simulink model "model_min_mine"  (R2018a)
settings: Solver=ode45  StartTime=0.0  StopTime=20  RelTol=1e-3
(part 1 of 10)
settings Model: Creator=Роман Стукан  LastModifiedBy=Роман Стукан

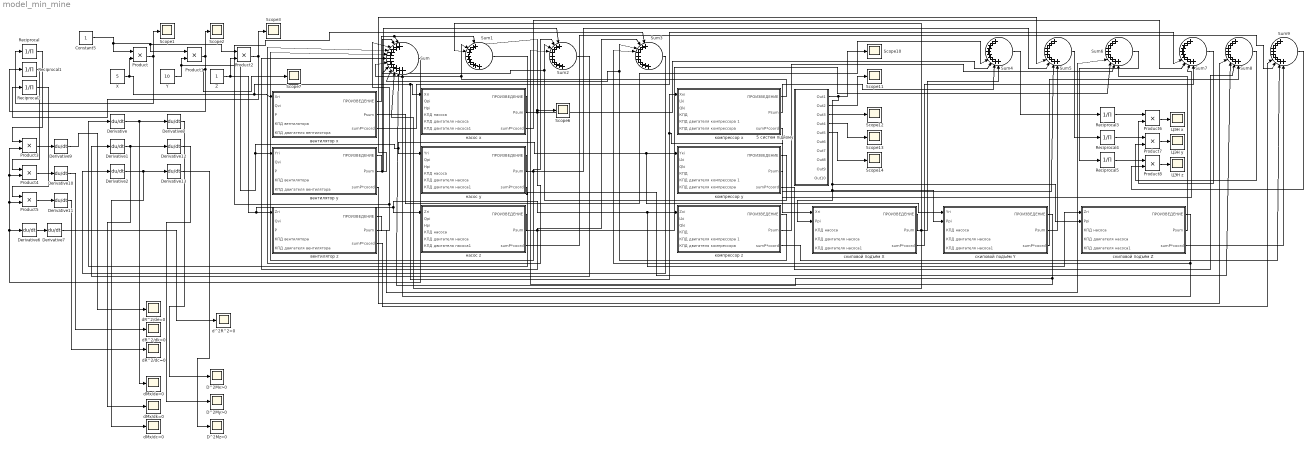
== system model_min_mine ==
  5 систем підйому : Subsystem
  Constant5 : Constant
  D^2Mx>0 : Scope
  D^2My>0 : Scope
  D^2Mz>0 : Scope
  Derivative{,1..2,6..13} (11 alike) : Derivative
  Product{,1..8} (9 alike) : Product
  Reciprocal{,1..5} (6 alike) : Product  Inputs=/  SaturateOnIntegerOverflow=on  RndMeth=Zero
  Scope{1..3,6..7,10..14} (10 alike) : Scope
  Sum : Sum  Inputs=|++++++++++++
  Sum{1..9} (9 alike) : Sum  Inputs=|++++++++++
  X : Constant  Value=5
  Y : Constant  Value=10
  Z : Constant
  dMx/dc=0 : Scope
  dMx/de=0 : Scope
  dMx/dk=0 : Scope
  dR^2/dc=0 : Scope
  dR^2/de=0 : Scope
  dR^2/dk=0 : Scope
  d^2R^2>0 : Scope
  ЦЭН x : Scope
  ЦЭН y : Scope
  ЦЭН z : Scope
  вентилятор x : Subsystem
  вентилятор y : Subsystem
  вентилятор z : Subsystem
  компрессор x : Subsystem
  компрессор y : Subsystem
  компрессор z : Subsystem
  насос x : Subsystem
  насос y : Subsystem
  насос z : Subsystem
  скиповой подъём Y : Subsystem
  скиповой подъём Z : Subsystem
  скиповой подъём Х : Subsystem
  wires:
  X/1 -> Product/2, скиповой подъём Х/1(Xri), компрессор x/1(Xкi), насос x/1(Xri), вентилятор x/1(Xri)
  Y/1 -> Product1/2, скиповой подъём Y/1(Yri), компрессор y/1(Yкi), насос y/1(Yri), вентилятор y/1(Yri)
  Z/1 -> Product2/2, скиповой подъём Z/1(Zri), компрессор z/1(Zкi), насос z/1(Zri), вентилятор z/1(Zri)
  вентилятор y/1(ПРОИЗВЕДЕНИЕ) -> Sum2/1, Sum/2
  вентилятор z/1(ПРОИЗВЕДЕНИЕ) -> Sum3/1, Sum/3
  насос x/1(ПРОИЗВЕДЕНИЕ) -> Scope6/1, Sum1/2, Sum/4
  насос y/1(ПРОИЗВЕДЕНИЕ) -> Sum2/2, Sum/5
  насос z/1(ПРОИЗВЕДЕНИЕ) -> Sum3/2, Sum/6
  вентилятор x/1(ПРОИЗВЕДЕНИЕ) -> Sum1/1, Sum/1
  Sum1/1 -> Derivative/1
  Sum2/1 -> Derivative1/1
  Sum3/1 -> Derivative2/1
  Constant5/1 -> Product2/1, Product1/1, Product/1
  Product/1 -> Scope1/1, Reciprocal/1
  Product1/1 -> Scope2/1, Reciprocal1/1, Scope7/1
  Product2/1 -> Scope3/1, Reciprocal2/1
  Reciprocal/1 -> Product3/1
  Reciprocal1/1 -> Product4/1
  Reciprocal2/1 -> Product5/1
  Sum/1 -> Derivative6/1, Product5/2, Product4/2, Product3/2
  Product5/1 -> Derivative11/1
  Product4/1 -> Derivative10/1
  Product3/1 -> Derivative9/1
  компрессор x/1(ПРОИЗВЕДЕНИЕ) -> Sum/7, Sum1/3
  компрессор y/1(ПРОИЗВЕДЕНИЕ) -> Sum/8, Sum2/3
  компрессор z/1(ПРОИЗВЕДЕНИЕ) -> Sum/9, Sum3/3
  Derivative9/1 -> dR^2/de=0/1
  Derivative10/1 -> dR^2/dk=0/1
  Derivative11/1 -> dR^2/dc=0/1
  5 систем підйому/2(Out2) -> Scope11/1
  5 систем підйому/3(Out3) -> Scope12/1
  5 систем підйому/4(Out4) -> Scope13/1
  5 систем підйому/5(Out5) -> Scope14/1
  5 систем підйому/1(Out1) -> скиповой подъём Z/2(Ррi), скиповой подъём Y/2(Ррi), скиповой подъём Х/2(Ррi), Scope10/1
  скиповой подъём Х/1(ПРОИЗВЕДЕНИЕ) -> Sum/10, Sum1/4
  скиповой подъём Z/1(ПРОИЗВЕДЕНИЕ) -> Sum/12, Sum3/4
  скиповой подъём Y/1(ПРОИЗВЕДЕНИЕ) -> Sum/11, Sum2/4
  Derivative6/1 -> Derivative7/1
  Derivative7/1 -> d^2R^2>0/1
  Derivative8/1 -> D^2Mx>0/1
  Derivative/1 -> Derivative8/1, dMx/de=0/1
  Derivative1/1 -> Derivative12/1, dMx/dk=0/1
  Derivative12/1 -> D^2My>0/1
  Derivative2/1 -> Derivative13/1, dMx/dc=0/1
  Derivative13/1 -> D^2Mz>0/1
  скиповой подъём Z/2(Psum) -> Sum6/10
  компрессор x/2(Psum) -> Sum4/9
  скиповой подъём Х/2(Psum) -> Sum4/10
  скиповой подъём Y/2(Psum) -> Sum5/10
  компрессор z/2(Psum) -> Sum6/9
  компрессор y/2(Psum) -> Sum5/9
  насос z/2(Psum) -> Sum6/8
  насос x/2(Psum) -> Sum4/8
  насос y/2(Psum) -> Sum5/8
  вентилятор z/2(Psum) -> Sum6/7
  вентилятор y/2(Psum) -> Sum5/7
  вентилятор x/2(Psum) -> Sum4/7
  Sum4/1 -> Reciprocal3/1
  Sum5/1 -> Reciprocal4/1
  Sum6/1 -> Reciprocal5/1
  Reciprocal3/1 -> Product6/1
  Reciprocal4/1 -> Product7/1
  Reciprocal5/1 -> Product8/1
  Product6/1 -> ЦЭН x/1
  Product7/1 -> ЦЭН y/1
  Product8/1 -> ЦЭН z/1
  скиповой подъём Z/3(sumP*coord) -> Sum9/10
  скиповой подъём Y/3(sumP*coord) -> Sum8/10
  скиповой подъём Х/3(sumP*coord) -> Sum7/10
  Sum7/1 -> Product6/2
  Sum8/1 -> Product7/2
  Sum9/1 -> Product8/2
  компрессор z/3(sumP*coord) -> Sum9/9
  компрессор y/3(sumP*coord) -> Sum8/9
  компрессор x/3(sumP*coord) -> Sum7/9
  насос z/3(sumP*coord) -> Sum9/8
  вентилятор x/3(sumP*coord) -> Sum7/7
  насос y/3(sumP*coord) -> Sum8/8
  насос x/3(sumP*coord) -> Sum7/8
  вентилятор y/3(sumP*coord) -> Sum8/7
  вентилятор z/3(sumP*coord) -> Sum9/7

== system model_min_mine/5 систем підйому ==
  1 : Subsystem
  2 : Subsystem
  3 : Subsystem
  4 : Subsystem
  6 : Subsystem
  Manual Switch{1..4,7} (5 alike) : ManualSwitch
  Out1 : Outport
  Out2 : Outport  Port=2
  Out3 : Outport  Port=3
  Out4 : Outport  Port=4
  Out5 : Outport  Port=5
  Out6 : Outport  Port=6
  Out7 : Outport  Port=7
  Out8 : Outport  Port=8
  Out9 : Outport  Port=9
  Out10 : Outport  Port=10
  wires:
  1/1(Out1) -> Manual Switch7/1
  Manual Switch7/1 -> Out1/1
  2/1(Out1) -> Manual Switch1/1
  3/1(Out1) -> Manual Switch2/1
  4/1(Out1) -> Manual Switch3/1
  6/1(Out1) -> Manual Switch4/1
  Manual Switch1/1 -> Out2/1
  Manual Switch2/1 -> Out3/1
  Manual Switch3/1 -> Out4/1
  Manual Switch4/1 -> Out5/1
  1/2(Out3) -> Out6/1
  2/2(Out3) -> Out7/1
  3/2(Out3) -> Out8/1
  4/2(Out3) -> Out9/1
  6/2(Out3) -> Out10/1

== system model_min_mine/вентилятор x ==
  Xri : Inport
  Qvi : Inport  Port=2
  P : Inport  Port=3
  КПД вентилятора : Inport  Port=4
  КПД двигателя вентилятора : Inport  Port=5
  Constant : Constant  Value=3000
  Constant1 : Constant  Value=284
  Constant2 : Constant  Value=1000
  Constant3 : Constant  Value=0.6
  Constant4 : Constant  Value=0.9
  Constant5 : Constant
  Math Function : Math  Operator=square  SaturateOnIntegerOverflow=on
  Product{,3..5} (4 alike) : Product
  Product1 : Product  Inputs=3
  Product2 : Product  Inputs=3
  Reciprocal : Product  Inputs=/  SaturateOnIntegerOverflow=on  RndMeth=Zero
  Scope6 : Scope
  Scope7 : Scope
  Sum : Sum  Inputs=|-++
  Sum{1..4} (4 alike) : Sum  Inputs=|++
  Transfer Fcn : TransferFcn  Denominator=[0.5 1]
  Xгвуi : Constant  Value=10
  ПРОИЗВЕДЕНИЕ : Outport
  Psum : Outport  Port=2
  sumP*coord : Outport  Port=3
  wires:
  Sum1/1 -> Product/1
  Product1/1 -> Reciprocal/1
  Constant/1 -> Transfer Fcn/1
  Product/1 -> Product4/1, Product2/1
  Constant2/1 -> Product1/1
  Reciprocal/1 -> Product4/2, Product2/2
  Math Function/1 -> Product3/2
  Constant3/1 -> Sum3/1
  Sum3/1 -> Product1/2
  Constant4/1 -> Sum4/1
  КПД вентилятора/1 -> Sum3/2
  Sum4/1 -> Product1/3
  Sum2/1 -> Product/2
  Xгвуi/1 -> Product5/2, Sum/2
  КПД двигателя вентилятора/1 -> Sum4/2
  Sum/1 -> Math Function/1
  Constant1/1 -> Sum2/1
  Product3/1 -> ПРОИЗВЕДЕНИЕ/1
  Xri/1 -> Sum/1
  Qvi/1 -> Sum1/2
  P/1 -> Sum2/2
  Product2/1 -> Scope6/1, Scope7/1, Product3/1
  Product4/1 -> Product5/1, Psum/1
  Constant5/1 -> Product2/3
  Product5/1 -> sumP*coord/1
  Transfer Fcn/1 -> Sum1/1

== system model_min_mine/вентилятор y ==
  Yri : Inport
  Qvi : Inport  Port=2
  P : Inport  Port=3
  КПД вентилятора : Inport  Port=4
  КПД двигателя вентилятора : Inport  Port=5
  Constant : Constant  Value=3000
  Constant1 : Constant  Value=284
  Constant2 : Constant  Value=1000
  Constant3 : Constant  Value=0.6
  Constant4 : Constant  Value=0.9
  Constant5 : Constant
  Math Function : Math  Operator=square  SaturateOnIntegerOverflow=on
  Product{,3..5} (4 alike) : Product
  Product1 : Product  Inputs=3
  Product2 : Product  Inputs=3
  Reciprocal : Product  Inputs=/  SaturateOnIntegerOverflow=on  RndMeth=Zero
  Sum : Sum  Inputs=|-++
  Sum{1..4} (4 alike) : Sum  Inputs=|++
  Transfer Fcn : TransferFcn  Denominator=[0.5 1]
  Yгвуi : Constant  Value=5
  ПРОИЗВЕДЕНИЕ : Outport
  Psum : Outport  Port=2
  sumP*coord : Outport  Port=3
  wires:
  Sum1/1 -> Product/1
  Product1/1 -> Reciprocal/1
  Constant/1 -> Transfer Fcn/1
  Product/1 -> Product4/1, Product2/1
  Constant2/1 -> Product1/1
  Reciprocal/1 -> Product4/2, Product2/2
  Math Function/1 -> Product3/2
  Constant5/1 -> Product2/3
  Constant3/1 -> Sum3/1
  Sum3/1 -> Product1/2
  Constant4/1 -> Sum4/1
  КПД вентилятора/1 -> Sum3/2
  Sum4/1 -> Product1/3
  Sum2/1 -> Product/2
  Product2/1 -> Product3/1
  КПД двигателя вентилятора/1 -> Sum4/2
  Sum/1 -> Math Function/1
  Constant1/1 -> Sum2/1
  Product3/1 -> ПРОИЗВЕДЕНИЕ/1
  Yri/1 -> Sum/1
  Qvi/1 -> Sum1/2
  P/1 -> Sum2/2
  Product4/1 -> Product5/1, Psum/1
  Yгвуi/1 -> Product5/2, Sum/2
  Product5/1 -> sumP*coord/1
  Transfer Fcn/1 -> Sum1/1

== system model_min_mine/вентилятор z ==
  Zri : Inport
  Qvi : Inport  Port=2
  P : Inport  Port=3
  КПД вентилятора : Inport  Port=4
  КПД двигателя вентилятора : Inport  Port=5
  Constant : Constant  Value=3000
  Constant1 : Constant  Value=284
  Constant2 : Constant  Value=1000
  Constant3 : Constant  Value=0.6
  Constant4 : Constant  Value=0.9
  Constant5 : Constant
  Math Function : Math  Operator=square  SaturateOnIntegerOverflow=on
  Product{,3..5} (4 alike) : Product
  Product1 : Product  Inputs=3
  Product2 : Product  Inputs=3
  Reciprocal : Product  Inputs=/  SaturateOnIntegerOverflow=on  RndMeth=Zero
  Sum : Sum  Inputs=|-++
  Sum{1..4} (4 alike) : Sum  Inputs=|++
  Transfer Fcn : TransferFcn  Denominator=[0.5 1]
  Zгвуi : Constant
  ПРОИЗВЕДЕНИЕ : Outport
  Psum : Outport  Port=2
  sumP*coord : Outport  Port=3
  wires:
  Sum1/1 -> Product/1
  Product1/1 -> Reciprocal/1
  Constant/1 -> Transfer Fcn/1
  Product/1 -> Product4/1, Product2/1
  Constant2/1 -> Product1/1
  Reciprocal/1 -> Product4/2, Product2/2
  Math Function/1 -> Product3/2
  Constant5/1 -> Product2/3
  Constant3/1 -> Sum3/1
  Sum3/1 -> Product1/2
  Constant4/1 -> Sum4/1
  КПД вентилятора/1 -> Sum3/2
  Sum4/1 -> Product1/3
  Sum2/1 -> Product/2
  Product2/1 -> Product3/1
  КПД двигателя вентилятора/1 -> Sum4/2
  Sum/1 -> Math Function/1
  Constant1/1 -> Sum2/1
  Product3/1 -> ПРОИЗВЕДЕНИЕ/1
  Zri/1 -> Sum/1
  Qvi/1 -> Sum1/2
  P/1 -> Sum2/2
  Product4/1 -> Product5/1, Psum/1
  Zгвуi/1 -> Product5/2, Sum/2
  Product5/1 -> sumP*coord/1
  Transfer Fcn/1 -> Sum1/1

== system model_min_mine/компрессор x ==
  Xкi : Inport
  Lki : Inport  Port=2
  Qki : Inport  Port=3
  "КПД " : Inport  Port=4
  КПД двигателя компрессора 1 : Inport  Port=5
  КПД двигателя компрессора : Inport  Port=6
  Constant : Constant  Value=200
  Constant1 : Constant  Value=150
  Constant2 : Constant  Value=60
  Constant3 : Constant  Value=0.6
  Constant4 : Constant  Value=0.9
  Constant5 : Constant  Value=0.9
  Constant6 : Constant  Value=102
  Constant7 : Constant
  Constant8 : Constant  Value=1.1
  Math Function : Math  Operator=square  SaturateOnIntegerOverflow=on
  Product : Product  Inputs=3
  Product1 : Product  Inputs=5
  Product2 : Product  Inputs=3
  Product3 : Product
  Product4 : Product
  Product5 : Product
  Reciprocal : Product  Inputs=/  SaturateOnIntegerOverflow=on  RndMeth=Zero
  Scope7 : Scope
  Sum : Sum  Inputs=|-++
  Sum{1..5} (5 alike) : Sum  Inputs=|++
  Transfer Fcn : TransferFcn  Denominator=[0.3 1]
  Xкомпресора : Constant  Value=40
  ПРОИЗВЕДЕНИЕ : Outport
  Psum : Outport  Port=2
  sumP*coord : Outport  Port=3
  wires:
  Sum1/1 -> Product/1
  Product1/1 -> Reciprocal/1
  Constant/1 -> Transfer Fcn/1
  Product/1 -> Product4/2, Product2/1
  Constant2/1 -> Product1/1
  Reciprocal/1 -> Product4/1, Product2/2
  Math Function/1 -> Product3/2
  Constant7/1 -> Product2/3
  Constant3/1 -> Sum3/1
  Sum3/1 -> Product1/2
  Constant4/1 -> Sum4/1
  "КПД "/1 -> Sum3/2
  Sum4/1 -> Product1/3
  Sum2/1 -> Product/2
  Product2/1 -> Scope7/1, Product3/1
  КПД двигателя компрессора 1/1 -> Sum4/2
  Sum/1 -> Math Function/1
  Constant1/1 -> Sum2/1
  Product3/1 -> ПРОИЗВЕДЕНИЕ/1
  Xкi/1 -> Sum/1
  Lki/1 -> Sum1/2
  Qki/1 -> Sum2/2
  Constant5/1 -> Sum5/1
  Sum5/1 -> Product1/5
  Constant6/1 -> Product1/4
  Constant8/1 -> Product/3
  КПД двигателя компрессора/1 -> Sum5/2
  Product4/1 -> Product5/1, Psum/1
  Xкомпресора/1 -> Product5/2, Sum/2
  Product5/1 -> sumP*coord/1
  Transfer Fcn/1 -> Sum1/1

== system model_min_mine/компрессор y ==
  Yкi : Inport
  Lki : Inport  Port=2
  Qki : Inport  Port=3
  "КПД " : Inport  Port=4
  КПД двигателя компрессора 1 : Inport  Port=5
  КПД двигателя компрессора : Inport  Port=6
  Constant : Constant  Value=200
  Constant1 : Constant  Value=150
  Constant2 : Constant  Value=60
  Constant3 : Constant  Value=0.6
  Constant4 : Constant  Value=0.9
  Constant5 : Constant  Value=0.9
  Constant6 : Constant  Value=102
  Constant7 : Constant
  Constant8 : Constant  Value=1.1
  Math Function : Math  Operator=square  SaturateOnIntegerOverflow=on
  Product : Product  Inputs=3
  Product1 : Product  Inputs=5
  Product2 : Product  Inputs=3
  Product3 : Product
  Product4 : Product
  Product5 : Product
  Reciprocal : Product  Inputs=/  SaturateOnIntegerOverflow=on  RndMeth=Zero
  Sum : Sum  Inputs=|-++
  Sum{1..5} (5 alike) : Sum  Inputs=|++
  Transfer Fcn : TransferFcn  Denominator=[0.3 1]
  Yкомпресора : Constant  Value=140
  ПРОИЗВЕДЕНИЕ : Outport
  Psum : Outport  Port=2
  sumP*coord : Outport  Port=3
  wires:
  Sum1/1 -> Product/1
  Product1/1 -> Reciprocal/1
  Constant/1 -> Transfer Fcn/1
  Product/1 -> Product4/2, Product2/1
  Constant2/1 -> Product1/1
  Reciprocal/1 -> Product4/1, Product2/2
  Math Function/1 -> Product3/2
  Constant7/1 -> Product2/3
  Constant3/1 -> Sum3/1
  Sum3/1 -> Product1/2
  Constant4/1 -> Sum4/1
  "КПД "/1 -> Sum3/2
  Sum4/1 -> Product1/3
  Sum2/1 -> Product/2
  Product2/1 -> Product3/1
  КПД двигателя компрессора 1/1 -> Sum4/2
  Sum/1 -> Math Function/1
  Constant1/1 -> Sum2/1
  Product3/1 -> ПРОИЗВЕДЕНИЕ/1
  Yкi/1 -> Sum/1
  Lki/1 -> Sum1/2
  Qki/1 -> Sum2/2
  Constant5/1 -> Sum5/1
  Sum5/1 -> Product1/5
  Constant6/1 -> Product1/4
  Constant8/1 -> Product/3
  КПД двигателя компрессора/1 -> Sum5/2
  Product4/1 -> Product5/1, Psum/1
  Yкомпресора/1 -> Product5/2, Sum/2
  Product5/1 -> sumP*coord/1
  Transfer Fcn/1 -> Sum1/1

== system model_min_mine/компрессор z ==
  Zкi : Inport
  Lki : Inport  Port=2
  Qki : Inport  Port=3
  "КПД " : Inport  Port=4
  КПД двигателя компрессора 1 : Inport  Port=5
  КПД двигателя компрессора : Inport  Port=6
  Constant : Constant  Value=200
  Constant1 : Constant  Value=150
  Constant2 : Constant  Value=60
  Constant3 : Constant  Value=0.6
  Constant4 : Constant  Value=0.9
  Constant5 : Constant  Value=0.9
  Constant6 : Constant  Value=102
  Constant7 : Constant
  Constant8 : Constant  Value=1.1
  Math Function : Math  Operator=square  SaturateOnIntegerOverflow=on
  Product : Product  Inputs=3
  Product1 : Product  Inputs=5
  Product2 : Product  Inputs=3
  Product3 : Product
  Product4 : Product
  Product5 : Product
  Reciprocal : Product  Inputs=/  SaturateOnIntegerOverflow=on  RndMeth=Zero
  Sum : Sum  Inputs=|-++
  Sum{1..5} (5 alike) : Sum  Inputs=|++
  Transfer Fcn : TransferFcn  Denominator=[0.3 1]
  Zкомпресора : Constant  Value=2
  ПРОИЗВЕДЕНИЕ : Outport
  Psum : Outport  Port=2
  sumP*coord : Outport  Port=3
  wires:
  Sum1/1 -> Product/1
  Product1/1 -> Reciprocal/1
  Constant/1 -> Transfer Fcn/1
  Product/1 -> Product4/2, Product2/1
  Constant2/1 -> Product1/1
  Reciprocal/1 -> Product4/1, Product2/2
  Math Function/1 -> Product3/2
  Constant7/1 -> Product2/3
  Constant3/1 -> Sum3/1
  Sum3/1 -> Product1/2
  Constant4/1 -> Sum4/1
  "КПД "/1 -> Sum3/2
  Sum4/1 -> Product1/3
  Sum2/1 -> Product/2
  Product2/1 -> Product3/1
  КПД двигателя компрессора 1/1 -> Sum4/2
  Sum/1 -> Math Function/1
  Constant1/1 -> Sum2/1
  Product3/1 -> ПРОИЗВЕДЕНИЕ/1
  Zкi/1 -> Sum/1
  Lki/1 -> Sum1/2
  Qki/1 -> Sum2/2
  Constant5/1 -> Sum5/1
  Sum5/1 -> Product1/5
  Constant6/1 -> Product1/4
  Constant8/1 -> Product/3
  КПД двигателя компрессора/1 -> Sum5/2
  Product4/1 -> Product5/1, Psum/1
  Zкомпресора/1 -> Product5/2, Sum/2
  Product5/1 -> sumP*coord/1
  Transfer Fcn/1 -> Sum1/1

== system model_min_mine/насос x ==
  Xri : Inport
  Qрi : Inport  Port=2
  Hpi : Inport  Port=3
  КПД насоса : Inport  Port=4
  КПД двигателя насоса : Inport  Port=5
  КПД двигателя насоса1 : Inport  Port=6
  Constant : Constant  Value=300
  Constant1 : Constant  Value=600
  Constant2 : Constant  Value=1000
  Constant3 : Constant  Value=0.6
  Constant4 : Constant  Value=0.9
  Constant5 : Constant  Value=0.9
  Constant6 : Constant  Value=3600
  Constant7 : Constant
  Constant8 : Constant  Value=9.81
  Math Function : Math  Operator=square  SaturateOnIntegerOverflow=on
  Product : Product  Inputs=4
  Product1 : Product  Inputs=5
  Product2 : Product  Inputs=3
  Product3 : Product
  Product4 : Product
  Product5 : Product
  Reciprocal : Product  Inputs=/  SaturateOnIntegerOverflow=on  RndMeth=Zero
  Scope7 : Scope
  Sum : Sum  Inputs=|-++
  Sum{1..5} (5 alike) : Sum  Inputs=|++
  Transfer Fcn : TransferFcn  Denominator=[0.02 1]
  Xгводоотливi : Constant  Value=100
  ро : Constant  Value=1200
  ПРОИЗВЕДЕНИЕ : Outport
  Psum : Outport  Port=2
  sumP*coord : Outport  Port=3
  wires:
  Sum1/1 -> Product/1
  Product1/1 -> Reciprocal/1
  Constant/1 -> Transfer Fcn/1
  Product/1 -> Product4/1, Product2/1
  Constant2/1 -> Product1/1
  Reciprocal/1 -> Product4/2, Product2/2
  Math Function/1 -> Product3/2
  Constant7/1 -> Product2/3
  Constant3/1 -> Sum3/1
  Sum3/1 -> Product1/2
  Constant4/1 -> Sum4/1
  КПД насоса/1 -> Sum3/2
  Sum4/1 -> Product1/3
  Sum2/1 -> Product/2
  Product2/1 -> Scope7/1, Product3/1
  КПД двигателя насоса/1 -> Sum4/2
  Sum/1 -> Math Function/1
  Constant1/1 -> Sum2/1
  Product3/1 -> ПРОИЗВЕДЕНИЕ/1
  Xri/1 -> Sum/1
  Qрi/1 -> Sum1/2
  Hpi/1 -> Sum2/2
  Constant5/1 -> Sum5/1
  Sum5/1 -> Product1/5
  Constant6/1 -> Product1/4
  ро/1 -> Product/4
  Constant8/1 -> Product/3
  КПД двигателя насоса1/1 -> Sum5/2
  Product4/1 -> Product5/1, Psum/1
  Xгводоотливi/1 -> Product5/2, Sum/2
  Product5/1 -> sumP*coord/1
  Transfer Fcn/1 -> Sum1/1

== system model_min_mine/насос y ==
  Yri : Inport
  Qрi : Inport  Port=2
  Hpi : Inport  Port=3
  КПД насоса : Inport  Port=4
  КПД двигателя насоса : Inport  Port=5
  КПД двигателя насоса1 : Inport  Port=6
  Constant : Constant  Value=300
  Constant1 : Constant  Value=600
  Constant2 : Constant  Value=1000
  Constant3 : Constant  Value=0.6
  Constant4 : Constant  Value=0.9
  Constant5 : Constant  Value=0.9
  Constant6 : Constant  Value=3600
  Constant7 : Constant
  Constant8 : Constant  Value=9.81
  Math Function : Math  Operator=square  SaturateOnIntegerOverflow=on
  Product : Product  Inputs=4
  Product1 : Product  Inputs=5
  Product2 : Product  Inputs=3
  Product3 : Product
  Product4 : Product
  Product5 : Product
  Reciprocal : Product  Inputs=/  SaturateOnIntegerOverflow=on  RndMeth=Zero
  Sum : Sum  Inputs=|-++
  Sum{1..5} (5 alike) : Sum  Inputs=|++
  Transfer Fcn : TransferFcn  Denominator=[0.02 1]
  Yгводоотливi : Constant  Value=20
  ро : Constant  Value=1200
  ПРОИЗВЕДЕНИЕ : Outport
  Psum : Outport  Port=2
  sumP*coord : Outport  Port=3
  wires:
  Sum1/1 -> Product/1
  Product1/1 -> Reciprocal/1
  Constant/1 -> Transfer Fcn/1
  Product/1 -> Product4/1, Product2/1
  Constant2/1 -> Product1/1
  Reciprocal/1 -> Product4/2, Product2/2
  Math Function/1 -> Product3/2
  Constant7/1 -> Product2/3
  Constant3/1 -> Sum3/1
  Sum3/1 -> Product1/2
  Constant4/1 -> Sum4/1
  КПД насоса/1 -> Sum3/2
  Sum4/1 -> Product1/3
  Sum2/1 -> Product/2
  Product2/1 -> Product3/1
  КПД двигателя насоса/1 -> Sum4/2
  Sum/1 -> Math Function/1
  Constant1/1 -> Sum2/1
  Product3/1 -> ПРОИЗВЕДЕНИЕ/1
  Yri/1 -> Sum/1
  Qрi/1 -> Sum1/2
  Hpi/1 -> Sum2/2
  Constant5/1 -> Sum5/1
  Sum5/1 -> Product1/5
  Constant6/1 -> Product1/4
  ро/1 -> Product/4
  Constant8/1 -> Product/3
  КПД двигателя насоса1/1 -> Sum5/2
  Product4/1 -> Product5/1, Psum/1
  Yгводоотливi/1 -> Product5/2, Sum/2
  Product5/1 -> sumP*coord/1
  Transfer Fcn/1 -> Sum1/1

== system model_min_mine/насос z ==
  Zri : Inport
  Qрi : Inport  Port=2
  Hpi : Inport  Port=3
  КПД насоса : Inport  Port=4
  КПД двигателя насоса : Inport  Port=5
  КПД двигателя насоса1 : Inport  Port=6
  Constant : Constant  Value=300
  Constant1 : Constant  Value=600
  Constant2 : Constant  Value=1000
  Constant3 : Constant  Value=0.6
  Constant4 : Constant  Value=0.9
  Constant5 : Constant  Value=0.9
  Constant6 : Constant  Value=3600
  Constant7 : Constant
  Constant8 : Constant  Value=9.81
  Math Function : Math  Operator=square  SaturateOnIntegerOverflow=on
  Product : Product  Inputs=4
  Product1 : Product  Inputs=5
  Product2 : Product  Inputs=3
  Product3 : Product
  Product4 : Product
  Product5 : Product
  Reciprocal : Product  Inputs=/  SaturateOnIntegerOverflow=on  RndMeth=Zero
  Sum : Sum  Inputs=|-++
  Sum{1..5} (5 alike) : Sum  Inputs=|++
  Transfer Fcn : TransferFcn  Denominator=[0.02 1]
  Zгводоотливi : Constant  Value=-500
  ро : Constant  Value=1200
  ПРОИЗВЕДЕНИЕ : Outport
  Psum : Outport  Port=2
  sumP*coord : Outport  Port=3
  wires:
  Sum1/1 -> Product/1
  Product1/1 -> Reciprocal/1
  Constant/1 -> Transfer Fcn/1
  Product/1 -> Product4/2, Product2/1
  Constant2/1 -> Product1/1
  Reciprocal/1 -> Product4/1, Product2/2
  Math Function/1 -> Product3/2
  Constant7/1 -> Product2/3
  Constant3/1 -> Sum3/1
  Sum3/1 -> Product1/2
  Constant4/1 -> Sum4/1
  КПД насоса/1 -> Sum3/2
  Sum4/1 -> Product1/3
  Sum2/1 -> Product/2
  Product2/1 -> Product3/1
  КПД двигателя насоса/1 -> Sum4/2
  Sum/1 -> Math Function/1
  Constant1/1 -> Sum2/1
  Product3/1 -> ПРОИЗВЕДЕНИЕ/1
  Zri/1 -> Sum/1
  Qрi/1 -> Sum1/2
  Hpi/1 -> Sum2/2
  Constant5/1 -> Sum5/1
  Sum5/1 -> Product1/5
  Constant6/1 -> Product1/4
  ро/1 -> Product/4
  Constant8/1 -> Product/3
  КПД двигателя насоса1/1 -> Sum5/2
  Product4/1 -> Product5/1, Psum/1
  Zгводоотливi/1 -> Product5/2, Sum/2
  Product5/1 -> sumP*coord/1
  Transfer Fcn/1 -> Sum1/1

== system model_min_mine/скиповой подъём Y ==
  Yri : Inport
  Ррi : Inport  Port=2
  КПД насоса : Inport  Port=3
  КПД двигателя насоса : Inport  Port=4
  КПД двигателя насоса1 : Inport  Port=5
  Constant1 : Constant
  Constant2 : Constant  Value=3600
  Constant3 : Constant  Value=0.6
  Constant4 : Constant  Value=0.9
  Constant5 : Constant  Value=0.9
  Constant6 : Constant  Value=3600
  Math Function : Math  Operator=square  SaturateOnIntegerOverflow=on
  Product1 : Product  Inputs=5
  Product2 : Product  Inputs=3
  Product3 : Product
  Product4 : Product
  Product5 : Product
  Reciprocal : Product  Inputs=/  SaturateOnIntegerOverflow=on  RndMeth=Zero
  Sum : Sum  Inputs=|-++
  Sum3 : Sum  Inputs=|++
  Sum4 : Sum  Inputs=|++
  Sum5 : Sum  Inputs=|++
  Transfer Fcn : TransferFcn  Denominator=[0.1 1]
  Xподъёмаi : Constant  Value=200
  ПРОИЗВЕДЕНИЕ : Outport
  Psum : Outport  Port=2
  sumP*coord : Outport  Port=3
  wires:
  Product1/1 -> Reciprocal/1
  Constant2/1 -> Product1/1
  Reciprocal/1 -> Product4/1, Product2/2
  Math Function/1 -> Product3/2
  Constant1/1 -> Product2/3
  Constant3/1 -> Sum3/1
  Sum3/1 -> Product1/2
  Constant4/1 -> Sum4/1
  КПД насоса/1 -> Sum3/2
  Sum4/1 -> Product1/3
  Product2/1 -> Product3/1
  КПД двигателя насоса/1 -> Sum4/2
  Sum/1 -> Math Function/1
  Product3/1 -> ПРОИЗВЕДЕНИЕ/1
  Yri/1 -> Sum/1
  Constant5/1 -> Sum5/1
  Sum5/1 -> Product1/5
  Constant6/1 -> Product1/4
  КПД двигателя насоса1/1 -> Sum5/2
  Product4/1 -> Product5/1, Psum/1
  Xподъёмаi/1 -> Product5/2, Sum/2
  Product5/1 -> sumP*coord/1
  Ррi/1 -> Transfer Fcn/1
  Transfer Fcn/1 -> Product2/1, Product4/2

== system model_min_mine/скиповой подъём Z ==
  Zri : Inport
  Ррi : Inport  Port=2
  КПД насоса : Inport  Port=3
  КПД двигателя насоса : Inport  Port=4
  КПД двигателя насоса1 : Inport  Port=5
  Constant1 : Constant
  Constant2 : Constant  Value=3600
  Constant3 : Constant  Value=0.6
  Constant4 : Constant  Value=0.9
  Constant5 : Constant  Value=0.9
  Constant6 : Constant  Value=3600
  Math Function : Math  Operator=square  SaturateOnIntegerOverflow=on
  Product1 : Product  Inputs=5
  Product2 : Product  Inputs=3
  Product3 : Product
  Product4 : Product
  Product5 : Product
  Reciprocal : Product  Inputs=/  SaturateOnIntegerOverflow=on  RndMeth=Zero
  Sum : Sum  Inputs=|-++
  Sum3 : Sum  Inputs=|++
  Sum4 : Sum  Inputs=|++
  Sum5 : Sum  Inputs=|++
  Transfer Fcn : TransferFcn  Denominator=[0.1 1]
  Zодъёмаi : Constant  Value=0
  ПРОИЗВЕДЕНИЕ : Outport
  Psum : Outport  Port=2
  sumP*coord : Outport  Port=3
  wires:
  Product1/1 -> Reciprocal/1
  Constant2/1 -> Product1/1
  Reciprocal/1 -> Product4/1, Product2/2
  Math Function/1 -> Product3/2
  Constant1/1 -> Product2/3
  Constant3/1 -> Sum3/1
  Sum3/1 -> Product1/2
  Constant4/1 -> Sum4/1
  КПД насоса/1 -> Sum3/2
  Sum4/1 -> Product1/3
  Product2/1 -> Product3/1
  КПД двигателя насоса/1 -> Sum4/2
  Sum/1 -> Math Function/1
  Product3/1 -> ПРОИЗВЕДЕНИЕ/1
  Zri/1 -> Sum/1
  Constant5/1 -> Sum5/1
  Sum5/1 -> Product1/5
  Constant6/1 -> Product1/4
  КПД двигателя насоса1/1 -> Sum5/2
  Product4/1 -> Product5/1, Psum/1
  Zодъёмаi/1 -> Product5/2, Sum/2
  Product5/1 -> sumP*coord/1
  Ррi/1 -> Transfer Fcn/1
  Transfer Fcn/1 -> Product4/2, Product2/1

== system model_min_mine/скиповой подъём Х ==
  Xri : Inport
  Ррi : Inport  Port=2
  КПД насоса : Inport  Port=3
  КПД двигателя насоса : Inport  Port=4
  КПД двигателя насоса1 : Inport  Port=5
  Constant1 : Constant
  Constant2 : Constant  Value=3600
  Constant3 : Constant  Value=0.6
  Constant4 : Constant  Value=0.9
  Constant5 : Constant  Value=0.9
  Constant6 : Constant  Value=3600
  Math Function : Math  Operator=square  SaturateOnIntegerOverflow=on
  Product1 : Product  Inputs=5
  Product2 : Product  Inputs=3
  Product3 : Product
  Product4 : Product
  Product5 : Product
  Reciprocal : Product  Inputs=/  SaturateOnIntegerOverflow=on  RndMeth=Zero
  Scope7 : Scope
  Sum : Sum  Inputs=|-++
  Sum3 : Sum  Inputs=|++
  Sum4 : Sum  Inputs=|++
  Sum5 : Sum  Inputs=|++
  Transfer Fcn : TransferFcn  Denominator=[0.1 1]
  Xподъёмаi : Constant  Value=200
  ПРОИЗВЕДЕНИЕ : Outport
  Psum : Outport  Port=2
  sumP*coord : Outport  Port=3
  wires:
  Product1/1 -> Reciprocal/1
  Constant2/1 -> Product1/1
  Reciprocal/1 -> Product4/1, Product2/2
  Math Function/1 -> Product3/2
  Constant1/1 -> Product2/3
  Constant3/1 -> Sum3/1
  Sum3/1 -> Product1/2
  Constant4/1 -> Sum4/1
  КПД насоса/1 -> Sum3/2
  Sum4/1 -> Product1/3
  Product2/1 -> Scope7/1, Product3/1
  КПД двигателя насоса/1 -> Sum4/2
  Sum/1 -> Math Function/1
  Product3/1 -> ПРОИЗВЕДЕНИЕ/1
  Xri/1 -> Sum/1
  Constant5/1 -> Sum5/1
  Sum5/1 -> Product1/5
  Constant6/1 -> Product1/4
  КПД двигателя насоса1/1 -> Sum5/2
  Product4/1 -> Product5/1, Psum/1
  Xподъёмаi/1 -> Product5/2, Sum/2
  Product5/1 -> sumP*coord/1
  Ррi/1 -> Transfer Fcn/1
  Transfer Fcn/1 -> Product4/2, Product2/1

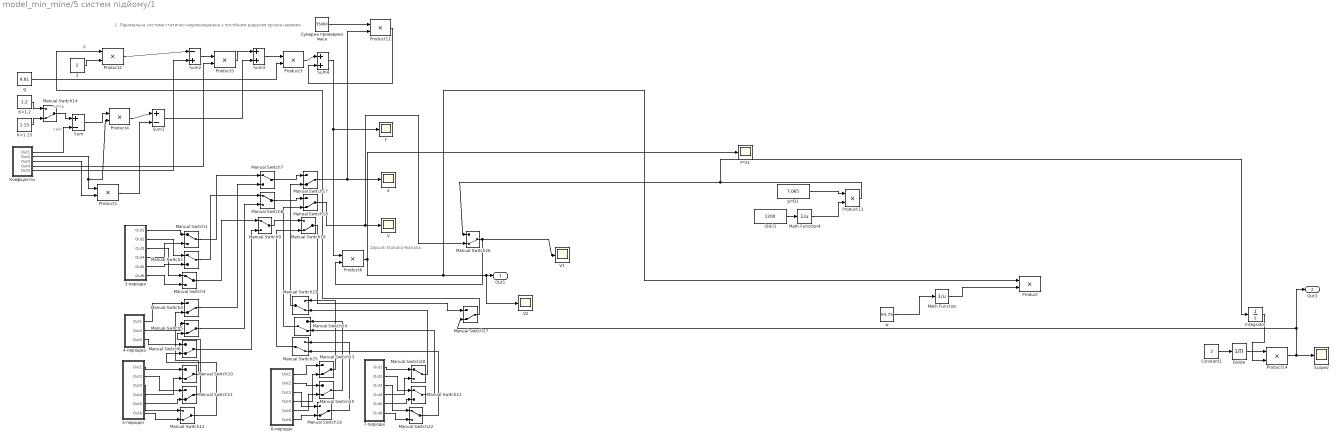
== system model_min_mine/5 систем підйому/1 ==
  note: 1. Піднімальна система статично неурівноважена з постійним
      | радіусом органа навивки
  note: Xi
  note: скіп
  note: кліть
  note: Zapusk Stukana Romana
  (60i)1 : Constant  Value=1200
  2 : Constant  Value=2
  3-періодні : Subsystem
  "4-періодна " : Subsystem
  5-періодні : Subsystem
  6-періодні : Subsystem
  7-періодні : Subsystem
  Constant1 : Constant  Value=2
  Divide : Product  Inputs=/
  F : Scope
  F*V1 : Scope
  Integrator : Integrator
  K=1.15 : Constant  Value=1.15
  K=1.2 : Constant  Value=1.2
  Manual Switch{1..3,7..9,20..22} (9 alike) : ManualSwitch
  Manual Switch{4..6,10..19,23..27} (18 alike) : ManualSwitch  CurrentSetting=0
  Math Function : Math  Operator=reciprocal  SaturateOnIntegerOverflow=on
  Math Function4 : Math  Operator=reciprocal  SaturateOnIntegerOverflow=on
  Product{,1..6,11,14} (9 alike) : Product  SaturateOnIntegerOverflow=on  OutDataTypeStr=Inherit: Same as first input
  Product13 : Product  Inputs=3  RndMeth=Zero
  Scope2 : Scope
  Sum : Sum  Inputs=|+-  SaturateOnIntegerOverflow=on
  Sum1 : Sum  Inputs=|+-  SaturateOnIntegerOverflow=on
  Sum2 : Sum  Inputs=|-+  SaturateOnIntegerOverflow=on
  Sum3 : Sum  Inputs=|++  SaturateOnIntegerOverflow=on
  Sum4 : Sum  Inputs=|++  SaturateOnIntegerOverflow=on
  V : Scope
  V1 : Scope
  V2 : Scope
  a : Scope
  g : Constant  Value=9.81
  pi*D1 : Constant  Value=7.065
  w : Constant  Value=93.75
  Коефіцієнти : Subsystem
  Сумарна приведена маса : Constant  Value=35000
  Out1 : Outport
  Out3 : Outport  Port=2
  wires:
  Manual Switch25/1 -> Manual Switch19/2
  Manual Switch24/1 -> Manual Switch18/2
  Manual Switch23/1 -> Manual Switch17/2
  Manual Switch16/1 -> Manual Switch25/1
  Manual Switch15/1 -> Manual Switch24/1
  Manual Switch13/1 -> Manual Switch23/1
  Manual Switch22/1 -> Manual Switch25/2
  Manual Switch21/1 -> Manual Switch24/2
  Manual Switch20/1 -> Manual Switch23/2
  Manual Switch8/1 -> Manual Switch18/1
  Manual Switch17/1 -> a/1, Product11/2
  Manual Switch7/1 -> Manual Switch17/1
  Manual Switch12/1 -> Manual Switch6/2
  Manual Switch11/1 -> Manual Switch5/2
  Manual Switch10/1 -> Manual Switch4/2
  Manual Switch6/1 -> Manual Switch9/2
  Manual Switch5/1 -> Manual Switch8/2
  Manual Switch4/1 -> Manual Switch7/2
  Manual Switch9/1 -> Manual Switch19/1
  Manual Switch2/1 -> Manual Switch8/1
  Manual Switch1/1 -> Manual Switch7/1
  Manual Switch3/1 -> Manual Switch9/1
  Product6/1 -> F*V1/1, V2/1, Out1/1, Product/1
  Product11/1 -> Sum4/2
  Сумарна приведена маса/1 -> Product11/1
  2/1 -> Product2/2
  Sum4/1 -> Product6/1, F/1
  Product3/1 -> Sum4/1
  Product5/1 -> Sum3/1
  Sum2/1 -> Product5/1
  Коефіцієнти/4(Out4) -> Product5/2
  g/1 -> Product3/2
  Sum3/1 -> Product3/1
  Sum1/1 -> Sum3/2
  Коефіцієнти/5(Out5) -> Sum2/2
  Product2/1 -> Sum2/1
  Product1/1 -> Sum1/2
  Product4/1 -> Sum1/1
  Коефіцієнти/3(Out3) -> Product1/2
  Коефіцієнти/2(Out2) -> Product4/2, Product1/1
  Sum/1 -> Product4/1
  Коефіцієнти/1(Out1) -> Sum/2
  Manual Switch14/1 -> Sum/1
  K=1.15/1 -> Manual Switch14/2
  K=1.2/1 -> Manual Switch14/1
  Manual Switch18/1 -> V/1, Manual Switch26/2
  3-періодні/1(Out1) -> Manual Switch1/1
  3-періодні/2(Out2) -> Manual Switch2/1
  3-періодні/3(Out3) -> Manual Switch3/1
  3-періодні/4(Out4) -> Manual Switch1/2
  3-періодні/5(Out5) -> Manual Switch2/2
  3-періодні/6(Out6) -> Manual Switch3/2
  "4-періодна "/1(Out1) -> Manual Switch4/1
  "4-періодна "/2(Out2) -> Manual Switch5/1
  "4-періодна "/3(Out3) -> Manual Switch6/1
  5-періодні/1(Out1) -> Manual Switch10/1
  5-періодні/2(Out2) -> Manual Switch11/1
  5-періодні/3(Out3) -> Manual Switch12/1
  5-періодні/4(Out4) -> Manual Switch10/2
  5-періодні/5(Out5) -> Manual Switch11/2
  5-періодні/6(Out6) -> Manual Switch12/2
  6-періодні/1(Out1) -> Manual Switch13/1
  6-періодні/2(Out2) -> Manual Switch15/1
  6-періодні/3(Out3) -> Manual Switch16/1
  6-періодні/4(Out4) -> Manual Switch13/2
  6-періодні/5(Out5) -> Manual Switch15/2
  6-періодні/6(Out6) -> Manual Switch16/2
  7-періодні/1(Out1) -> Manual Switch20/1
  7-періодні/2(Out2) -> Manual Switch21/1
  7-періодні/3(Out3) -> Manual Switch22/1
  7-періодні/4(Out4) -> Manual Switch20/2
  7-періодні/5(Out5) -> Manual Switch21/2
  7-періодні/6(Out6) -> Manual Switch22/2
  Math Function/1 -> Product/2
  w/1 -> Math Function/1
  Integrator/1 -> Product14/2
  Product14/1 -> Scope2/1, Out3/1, Manual Switch27/2
  Divide/1 -> Product14/1
  Constant1/1 -> Divide/1
  pi*D1/1 -> Product13/1
  (60i)1/1 -> Math Function4/1
  Math Function4/1 -> Product13/3
  Product13/1 -> Manual Switch26/1, Integrator/1
  Manual Switch26/1 -> Product6/2, V1/1
  Manual Switch27/1 -> Product2/1
  Manual Switch19/1 -> Manual Switch27/1

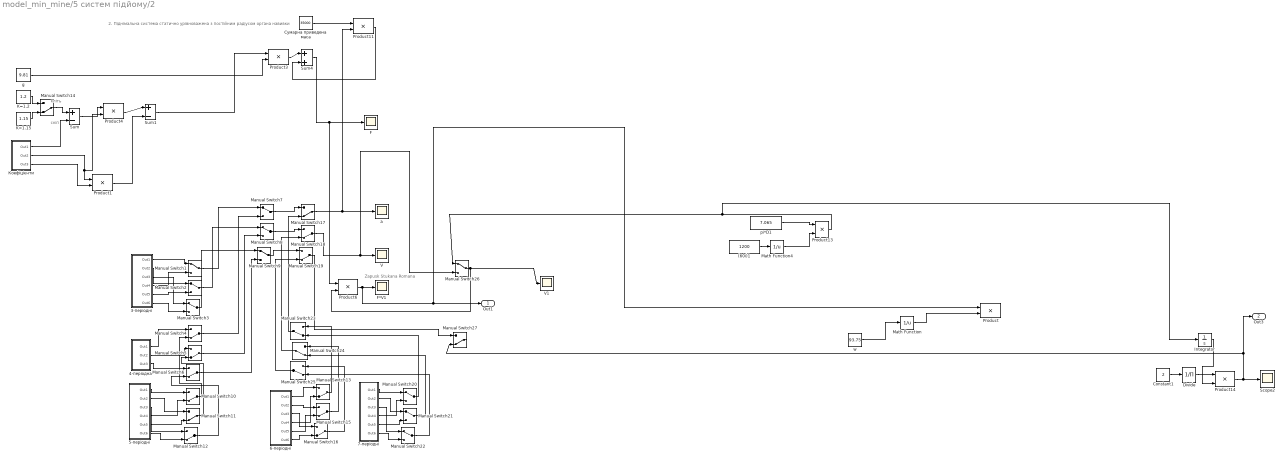
== system model_min_mine/5 систем підйому/2 ==
  note: кліть
  note: скіп
  note: 2. Піднімальна система статично урівноважена з постійним
      | радіусом органа навивки
  note: Zapusk Stukana Romana
  (60i)1 : Constant  Value=1200
  3-періодні : Subsystem
  "4-періодна " : Subsystem
  5-періодні : Subsystem
  6-періодні : Subsystem
  7-періодні : Subsystem
  Constant1 : Constant  Value=2
  Divide : Product  Inputs=/
  F : Scope
  F*V1 : Scope
  Integrator : Integrator
  K=1.15 : Constant  Value=1.15
  K=1.2 : Constant  Value=1.2
  Manual Switch{1..3,7..9,20..22,26} (10 alike) : ManualSwitch
  Manual Switch{4..6,10..19,23..25,27} (17 alike) : ManualSwitch  CurrentSetting=0
  Math Function : Math  Operator=reciprocal  SaturateOnIntegerOverflow=on
  Math Function4 : Math  Operator=reciprocal  SaturateOnIntegerOverflow=on
  Product{,1,3..4,6,11,14} (7 alike) : Product  SaturateOnIntegerOverflow=on  OutDataTypeStr=Inherit: Same as first input
  Product13 : Product  Inputs=3  RndMeth=Zero
  Scope2 : Scope
  Sum : Sum  Inputs=|+-  SaturateOnIntegerOverflow=on
  Sum1 : Sum  Inputs=|+-  SaturateOnIntegerOverflow=on
  Sum4 : Sum  Inputs=|++  SaturateOnIntegerOverflow=on
  V : Scope
  V1 : Scope
  a : Scope
  g : Constant  Value=9.81
  pi*D1 : Constant  Value=7.065
  w : Constant  Value=93.75
  Коефіцієнти : Subsystem
  Сумарна приведена маса : Constant  Value=35000
  Out1 : Outport
  Out3 : Outport  Port=2
  wires:
  K=1.2/1 -> Manual Switch14/1
  K=1.15/1 -> Manual Switch14/2
  Manual Switch14/1 -> Sum/1
  Коефіцієнти/1(Out1) -> Sum/2
  Sum/1 -> Product4/1
  Коефіцієнти/2(Out2) -> Product4/2, Product1/1
  Коефіцієнти/3(Out3) -> Product1/2
  Product4/1 -> Sum1/1
  Product1/1 -> Sum1/2
  g/1 -> Product3/2
  Product3/1 -> Sum4/1
  Sum4/1 -> F/1, Product6/1
  Сумарна приведена маса/1 -> Product11/1
  Product11/1 -> Sum4/2
  Sum1/1 -> Product3/1
  Manual Switch25/1 -> Manual Switch19/2
  Manual Switch24/1 -> Manual Switch18/2
  Manual Switch23/1 -> Manual Switch17/2
  Manual Switch16/1 -> Manual Switch25/1
  Manual Switch15/1 -> Manual Switch24/1
  Manual Switch13/1 -> Manual Switch23/1
  Manual Switch22/1 -> Manual Switch25/2
  Manual Switch21/1 -> Manual Switch24/2
  Manual Switch20/1 -> Manual Switch23/2
  Manual Switch8/1 -> Manual Switch18/1
  Manual Switch17/1 -> a/1, Product11/2
  Manual Switch7/1 -> Manual Switch17/1
  Manual Switch12/1 -> Manual Switch6/2
  Manual Switch11/1 -> Manual Switch5/2
  Manual Switch10/1 -> Manual Switch4/2
  Manual Switch6/1 -> Manual Switch9/2
  Manual Switch5/1 -> Manual Switch8/2
  Manual Switch4/1 -> Manual Switch7/2
  Manual Switch9/1 -> Manual Switch19/1
  Manual Switch2/1 -> Manual Switch8/1
  Manual Switch1/1 -> Manual Switch7/1
  Manual Switch3/1 -> Manual Switch9/1
  Product6/1 -> F*V1/1, Out1/1, Product/1
  Manual Switch18/1 -> V/1, Manual Switch26/2
  3-періодні/1(Out1) -> Manual Switch1/1
  3-періодні/2(Out2) -> Manual Switch2/1
  3-періодні/3(Out3) -> Manual Switch3/1
  3-періодні/4(Out4) -> Manual Switch1/2
  3-періодні/5(Out5) -> Manual Switch2/2
  3-періодні/6(Out6) -> Manual Switch3/2
  "4-періодна "/1(Out1) -> Manual Switch4/1
  "4-періодна "/2(Out2) -> Manual Switch5/1
  "4-періодна "/3(Out3) -> Manual Switch6/1
  5-періодні/1(Out1) -> Manual Switch10/1
  5-періодні/2(Out2) -> Manual Switch11/1
  5-періодні/3(Out3) -> Manual Switch12/1
  5-періодні/4(Out4) -> Manual Switch10/2
  5-періодні/5(Out5) -> Manual Switch11/2
  5-періодні/6(Out6) -> Manual Switch12/2
  6-періодні/1(Out1) -> Manual Switch13/1
  6-періодні/2(Out2) -> Manual Switch15/1
  6-періодні/3(Out3) -> Manual Switch16/1
  6-періодні/4(Out4) -> Manual Switch13/2
  6-періодні/5(Out5) -> Manual Switch15/2
  6-періодні/6(Out6) -> Manual Switch16/2
  7-періодні/1(Out1) -> Manual Switch20/1
  7-періодні/2(Out2) -> Manual Switch21/1
  7-періодні/3(Out3) -> Manual Switch22/1
  7-періодні/4(Out4) -> Manual Switch20/2
  7-періодні/5(Out5) -> Manual Switch21/2
  7-періодні/6(Out6) -> Manual Switch22/2
  Math Function/1 -> Product/2
  w/1 -> Math Function/1
  Integrator/1 -> Product14/2
  Product14/1 -> Scope2/1, Out3/1, Manual Switch27/2
  Divide/1 -> Product14/1
  Constant1/1 -> Divide/1
  pi*D1/1 -> Product13/1
  (60i)1/1 -> Math Function4/1
  Math Function4/1 -> Product13/3
  Product13/1 -> Manual Switch26/1, Integrator/1
  Manual Switch26/1 -> Product6/2, V1/1
  Manual Switch19/1 -> Manual Switch27/1

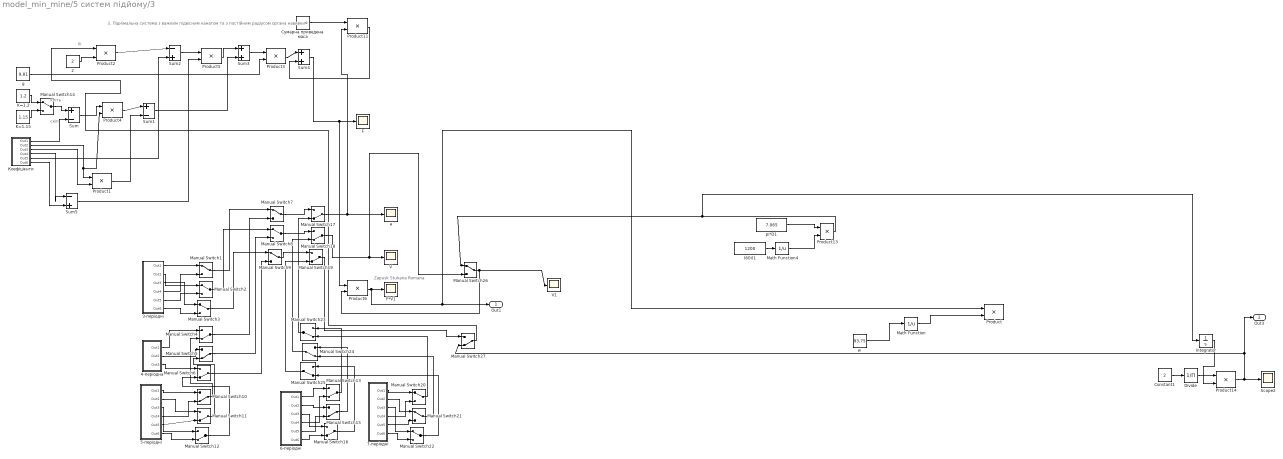
== system model_min_mine/5 систем підйому/3 ==
  note: кліть
  note: скіп
  note: Xi
  note: 3. Піднімальна система з важким підвісним канатом та з постійним
      | радіусом органа навивки
  note: Zapusk Stukana Romana
  (60i)1 : Constant  Value=1200
  2 : Constant  Value=2
  3-періодні : Subsystem
  "4-періодна " : Subsystem
  5-періодні : Subsystem
  6-періодні : Subsystem
  7-періодні : Subsystem
  Constant1 : Constant  Value=2
  Divide : Product  Inputs=/
  F : Scope
  F*V1 : Scope
  Integrator : Integrator
  K=1.15 : Constant  Value=1.15
  K=1.2 : Constant  Value=1.2
  Manual Switch{1..3,7..9,14,20..22,26} (11 alike) : ManualSwitch
  Manual Switch{4..6,10..13,15..19,23..25,27} (16 alike) : ManualSwitch  CurrentSetting=0
  Math Function : Math  Operator=reciprocal  SaturateOnIntegerOverflow=on
  Math Function4 : Math  Operator=reciprocal  SaturateOnIntegerOverflow=on
  Product{,1..6,11,14} (9 alike) : Product  SaturateOnIntegerOverflow=on  OutDataTypeStr=Inherit: Same as first input
  Product13 : Product  Inputs=3  RndMeth=Zero
  Scope2 : Scope
  Sum : Sum  Inputs=|+-  SaturateOnIntegerOverflow=on
  Sum1 : Sum  Inputs=|+-  SaturateOnIntegerOverflow=on
  Sum2 : Sum  Inputs=|-+  SaturateOnIntegerOverflow=on
  Sum3 : Sum  Inputs=|++  SaturateOnIntegerOverflow=on
  Sum4 : Sum  Inputs=|++  SaturateOnIntegerOverflow=on
  Sum5 : Sum  Inputs=|-+  SaturateOnIntegerOverflow=on
  V : Scope
  V1 : Scope
  a : Scope
  g : Constant  Value=9.81
  pi*D1 : Constant  Value=7.065
  w : Constant  Value=93.75
  Коефіцієнти : Subsystem
  Сумарна приведена маса : Constant  Value=35000
  Out1 : Outport
  Out3 : Outport  Port=2
  wires:
  K=1.2/1 -> Manual Switch14/1
  K=1.15/1 -> Manual Switch14/2
  Manual Switch14/1 -> Sum/1
  Коефіцієнти/1(Out1) -> Sum/2
  Sum/1 -> Product4/1
  Коефіцієнти/2(Out2) -> Product4/2, Product1/1
  Коефіцієнти/3(Out3) -> Product1/2
  Product4/1 -> Sum1/1
  Product1/1 -> Sum1/2
  Product2/1 -> Sum2/1
  Коефіцієнти/5(Out5) -> Sum2/2
  Sum1/1 -> Sum3/2
  Sum3/1 -> Product3/1
  g/1 -> Product3/2
  Коефіцієнти/4(Out4) -> Sum5/1
  Sum2/1 -> Product5/1
  Product5/1 -> Sum3/1
  Product3/1 -> Sum4/1
  Sum4/1 -> F/1, Product6/1
  2/1 -> Product2/2
  Сумарна приведена маса/1 -> Product11/1
  Product11/1 -> Sum4/2
  Коефіцієнти/6(Out6) -> Sum5/2
  Sum5/1 -> Product5/2
  Manual Switch25/1 -> Manual Switch19/2
  Manual Switch24/1 -> Manual Switch18/2
  Manual Switch23/1 -> Manual Switch17/2
  Manual Switch16/1 -> Manual Switch25/1
  Manual Switch15/1 -> Manual Switch24/1
  Manual Switch13/1 -> Manual Switch23/1
  Manual Switch22/1 -> Manual Switch25/2
  Manual Switch21/1 -> Manual Switch24/2
  Manual Switch20/1 -> Manual Switch23/2
  Manual Switch8/1 -> Manual Switch18/1
  Manual Switch17/1 -> a/1, Product11/2
  Manual Switch7/1 -> Manual Switch17/1
  Manual Switch12/1 -> Manual Switch6/2
  Manual Switch11/1 -> Manual Switch5/2
  Manual Switch10/1 -> Manual Switch4/2
  Manual Switch6/1 -> Manual Switch9/2
  Manual Switch5/1 -> Manual Switch8/2
  Manual Switch4/1 -> Manual Switch7/2
  Manual Switch9/1 -> Manual Switch19/1
  Manual Switch2/1 -> Manual Switch8/1
  Manual Switch1/1 -> Manual Switch7/1
  Manual Switch3/1 -> Manual Switch9/1
  Product6/1 -> F*V1/1, Out1/1, Product/1
  Manual Switch18/1 -> V/1, Manual Switch26/2
  3-періодні/1(Out1) -> Manual Switch1/1
  3-періодні/2(Out2) -> Manual Switch2/1
  3-періодні/3(Out3) -> Manual Switch3/1
  3-періодні/4(Out4) -> Manual Switch1/2
  3-періодні/5(Out5) -> Manual Switch2/2
  3-періодні/6(Out6) -> Manual Switch3/2
  "4-періодна "/1(Out1) -> Manual Switch4/1
  "4-періодна "/2(Out2) -> Manual Switch5/1
  "4-періодна "/3(Out3) -> Manual Switch6/1
  5-періодні/1(Out1) -> Manual Switch10/1
  5-періодні/2(Out2) -> Manual Switch11/1
  5-періодні/3(Out3) -> Manual Switch12/1
  5-періодні/4(Out4) -> Manual Switch10/2
  5-періодні/5(Out5) -> Manual Switch11/2
  5-періодні/6(Out6) -> Manual Switch12/2
  6-періодні/1(Out1) -> Manual Switch13/1
  6-періодні/2(Out2) -> Manual Switch15/1
  6-періодні/3(Out3) -> Manual Switch16/1
  6-періодні/4(Out4) -> Manual Switch13/2
  6-періодні/5(Out5) -> Manual Switch15/2
  6-періодні/6(Out6) -> Manual Switch16/2
  7-періодні/1(Out1) -> Manual Switch20/1
  7-періодні/2(Out2) -> Manual Switch21/1
  7-періодні/3(Out3) -> Manual Switch22/1
  7-періодні/4(Out4) -> Manual Switch20/2
  7-періодні/5(Out5) -> Manual Switch21/2
  7-періодні/6(Out6) -> Manual Switch22/2
  Math Function/1 -> Product/2
  w/1 -> Math Function/1
  Integrator/1 -> Product14/2
  Product14/1 -> Scope2/1, Out3/1, Manual Switch27/2
  Divide/1 -> Product14/1
  Constant1/1 -> Divide/1
  pi*D1/1 -> Product13/1
  (60i)1/1 -> Math Function4/1
  Math Function4/1 -> Product13/3
  Product13/1 -> Manual Switch26/1, Integrator/1
  Manual Switch26/1 -> Product6/2, V1/1
  Manual Switch27/1 -> Product2/1
  Manual Switch19/1 -> Manual Switch27/1

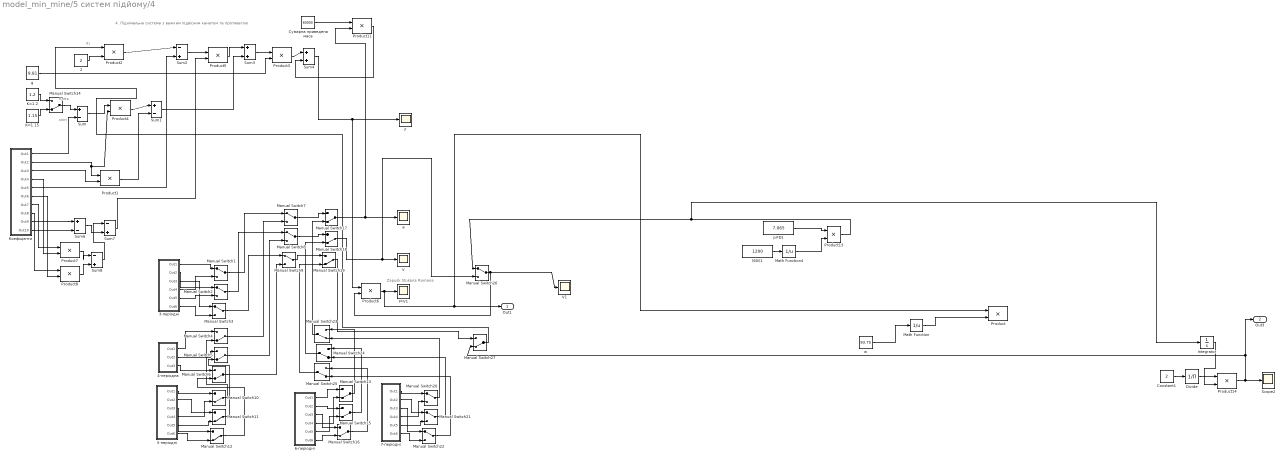
== system model_min_mine/5 систем підйому/4 ==
  note: кліть
  note: скіп
  note: Xi
  note: 4. Піднімальна система з важким підвісним канатом та противагою
  note: Zapusk Stukana Romana
  (60i)1 : Constant  Value=1200
  2 : Constant  Value=2
  3-періодні : Subsystem
  "4-періодна " : Subsystem
  5-періодні : Subsystem
  6-періодні : Subsystem
  7-періодні : Subsystem
  Constant1 : Constant  Value=2
  Divide : Product  Inputs=/
  F : Scope
  F*V1 : Scope
  Integrator : Integrator
  K=1.15 : Constant  Value=1.15
  K=1.2 : Constant  Value=1.2
  Manual Switch{1..3,7..9,20..22,26} (10 alike) : ManualSwitch
  Manual Switch{4..6,10..19,23..25,27} (17 alike) : ManualSwitch  CurrentSetting=0
  Math Function : Math  Operator=reciprocal  SaturateOnIntegerOverflow=on
  Math Function4 : Math  Operator=reciprocal  SaturateOnIntegerOverflow=on
  Product{,1..8,11,14} (11 alike) : Product  SaturateOnIntegerOverflow=on  OutDataTypeStr=Inherit: Same as first input
  Product13 : Product  Inputs=3  RndMeth=Zero
  Scope2 : Scope
  Sum : Sum  Inputs=|+-  SaturateOnIntegerOverflow=on
  Sum1 : Sum  Inputs=|+-  SaturateOnIntegerOverflow=on
  Sum2 : Sum  Inputs=|-+  SaturateOnIntegerOverflow=on
  Sum3 : Sum  Inputs=|++  SaturateOnIntegerOverflow=on
  Sum4 : Sum  Inputs=|++  SaturateOnIntegerOverflow=on
  Sum6 : Sum  Inputs=|+-  SaturateOnIntegerOverflow=on
  Sum7 : Sum  Inputs=|-+  SaturateOnIntegerOverflow=on
  Sum8 : Sum  Inputs=|-+  SaturateOnIntegerOverflow=on
  V : Scope
  V1 : Scope
  a : Scope
  g : Constant  Value=9.81
  pi*D1 : Constant  Value=7.065
  w : Constant  Value=93.75
  Коефіцієнти : Subsystem
  Сумарна приведена маса : Constant  Value=60000
  Out1 : Outport
  Out3 : Outport  Port=2
  wires:
  K=1.2/1 -> Manual Switch14/1
  K=1.15/1 -> Manual Switch14/2
  Manual Switch14/1 -> Sum/1
  Коефіцієнти/1(Out1) -> Sum/2
  Sum/1 -> Product4/1
  Коефіцієнти/2(Out2) -> Product4/2, Product1/1
  Коефіцієнти/3(Out3) -> Product1/2
  Product4/1 -> Sum1/1
  Product1/1 -> Sum1/2
  Product2/1 -> Sum2/1
  Коефіцієнти/5(Out5) -> Sum2/2
  Sum1/1 -> Sum3/2
  Sum3/1 -> Product3/1
  g/1 -> Product3/2
  Коефіцієнти/4(Out4) -> Product7/2
  Sum2/1 -> Product5/1
  Product5/1 -> Sum3/1
  Product3/1 -> Sum4/1
  Sum4/1 -> F/1, Product6/1
  2/1 -> Product2/2
  Сумарна приведена маса/1 -> Product11/1
  Product11/1 -> Sum4/2
  Коефіцієнти/6(Out6) -> Product8/2
  Коефіцієнти/9(Out9) -> Sum6/1
  Коефіцієнти/10(Out10) -> Sum6/2
  Sum6/1 -> Sum7/2
  Коефіцієнти/7(Out7) -> Product7/1
  Коефіцієнти/8(Out8) -> Product8/1
  Product8/1 -> Sum8/2
  Product7/1 -> Sum8/1
  Sum8/1 -> Sum7/1
  Sum7/1 -> Product5/2
  Manual Switch25/1 -> Manual Switch19/2
  Manual Switch24/1 -> Manual Switch18/2
  Manual Switch23/1 -> Manual Switch17/2
  Manual Switch16/1 -> Manual Switch25/1
  Manual Switch15/1 -> Manual Switch24/1
  Manual Switch13/1 -> Manual Switch23/1
  Manual Switch22/1 -> Manual Switch25/2
  Manual Switch21/1 -> Manual Switch24/2
  Manual Switch20/1 -> Manual Switch23/2
  Manual Switch8/1 -> Manual Switch18/1
  Manual Switch17/1 -> a/1, Product11/2
  Manual Switch7/1 -> Manual Switch17/1
  Manual Switch12/1 -> Manual Switch6/2
  Manual Switch11/1 -> Manual Switch5/2
  Manual Switch10/1 -> Manual Switch4/2
  Manual Switch6/1 -> Manual Switch9/2
  Manual Switch5/1 -> Manual Switch8/2
  Manual Switch4/1 -> Manual Switch7/2
  Manual Switch9/1 -> Manual Switch19/1
  Manual Switch2/1 -> Manual Switch8/1
  Manual Switch1/1 -> Manual Switch7/1
  Manual Switch3/1 -> Manual Switch9/1
  Product6/1 -> F*V1/1, Out1/1, Product/1
  Manual Switch18/1 -> V/1, Manual Switch26/2
  3-періодні/1(Out1) -> Manual Switch1/1
  3-періодні/2(Out2) -> Manual Switch2/1
  3-періодні/3(Out3) -> Manual Switch3/1
  3-періодні/4(Out4) -> Manual Switch1/2
  3-періодні/5(Out5) -> Manual Switch2/2
  3-періодні/6(Out6) -> Manual Switch3/2
  "4-періодна "/1(Out1) -> Manual Switch4/1
  "4-періодна "/2(Out2) -> Manual Switch5/1
  "4-періодна "/3(Out3) -> Manual Switch6/1
  5-періодні/1(Out1) -> Manual Switch10/1
  5-періодні/2(Out2) -> Manual Switch11/1
  5-періодні/3(Out3) -> Manual Switch12/1
  5-періодні/4(Out4) -> Manual Switch10/2
  5-періодні/5(Out5) -> Manual Switch11/2
  5-періодні/6(Out6) -> Manual Switch12/2
  6-періодні/1(Out1) -> Manual Switch13/1
  6-періодні/2(Out2) -> Manual Switch15/1
  6-періодні/3(Out3) -> Manual Switch16/1
  6-періодні/4(Out4) -> Manual Switch13/2
  6-періодні/5(Out5) -> Manual Switch15/2
  6-періодні/6(Out6) -> Manual Switch16/2
  7-періодні/1(Out1) -> Manual Switch20/1
  7-періодні/2(Out2) -> Manual Switch21/1
  7-періодні/3(Out3) -> Manual Switch22/1
  7-періодні/4(Out4) -> Manual Switch20/2
  7-періодні/5(Out5) -> Manual Switch21/2
  7-періодні/6(Out6) -> Manual Switch22/2
  Math Function/1 -> Product/2
  w/1 -> Math Function/1
  Integrator/1 -> Product14/2
  Product14/1 -> Scope2/1, Out3/1, Manual Switch27/2
  Divide/1 -> Product14/1
  Constant1/1 -> Divide/1
  pi*D1/1 -> Product13/1
  (60i)1/1 -> Math Function4/1
  Math Function4/1 -> Product13/3
  Product13/1 -> Manual Switch26/1, Integrator/1
  Manual Switch26/1 -> Product6/2, V1/1
  Manual Switch27/1 -> Product2/1
  Manual Switch19/1 -> Manual Switch27/1
